simulink model "lab04es01b_schema"  (R2021b)
settings: Solver=VariableStepAuto  StartTime=0.0  StopTime=20  RelTol=1e-3
undefined symbols (not defined in the file or in its folder): Kc3
libraries: cstblocks x2
settings Model: Creator=francescafornasier  LastModifiedBy=francescafornasier

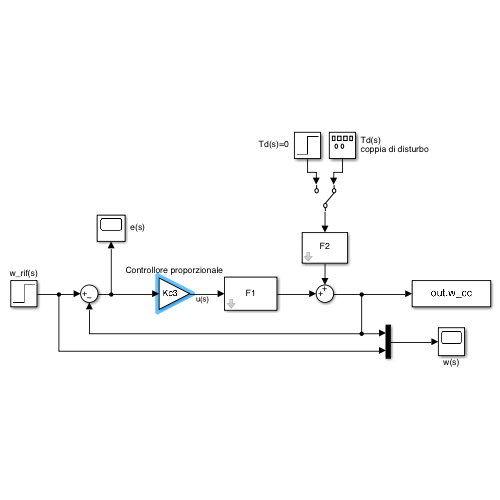
[thumbnail: Simulink's stored preview of the top-level diagram]
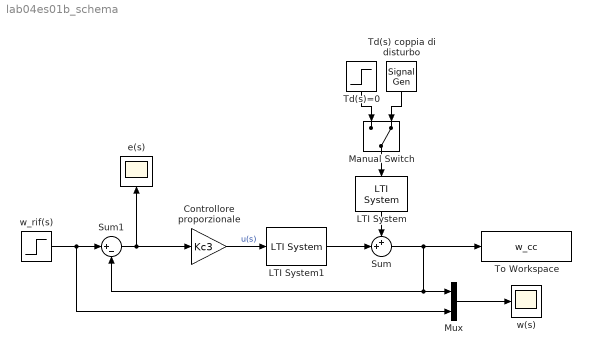
== system lab04es01b_schema ==
  Controllore proporzionale : Gain  Gain=Kc3
  LTI System : cstblocks/LTI System  sys=F2  IC=[]
  LTI System1 : cstblocks/LTI System  sys=F1  IC=[]
  Manual Switch : ManualSwitch  CurrentSetting=0
  Mux : Mux  Inputs=2
  Sum : Sum  Inputs=++|
  Sum1 : Sum  Inputs=|+-
  Td(s) coppia di disturbo : SignalGenerator  WaveForm=square  Amplitude=0.05  Frequency=0.1
  Td(s)=0 : Step  Time=0  After=0  SampleTime=0
  To Workspace : ToWorkspace  VariableName=w_cc  SaveFormat=Timeseries  SampleTime=-1
  e(s) : Scope
  w(s) : Scope
  w_rif(s) : Step  Time=0  SampleTime=0
  wires:
  LTI System/1 -> Sum/1
  LTI System1/1 -> Sum/2
  Manual Switch/1 -> LTI System/1
  w_rif(s)/1 -> Mux/2, Sum1/1
  Td(s)=0/1 -> Manual Switch/1
  Controllore proporzionale/1 -> LTI System1/1  "u(s)"
  Sum1/1 -> Controllore proporzionale/1, e(s)/1
  Mux/1 -> w(s)/1
  Sum/1 -> Mux/1, Sum1/2, To Workspace/1
  Td(s) coppia di disturbo/1 -> Manual Switch/2
